simulink model "LoRaWAN_withoutGolay"  (R2021a)
settings: Solver=VariableStepAuto  StartTime=0.0  StopTime=1  RelTol=1e-3
libraries: commdigbbndcpm2 x2, commchan3 x1, commsink2 x1, commutil2 x1, commrflib2 x1, commrandsrc3 x1
settings Model: Creator=saivittalb  LastModifiedBy=saivittalb

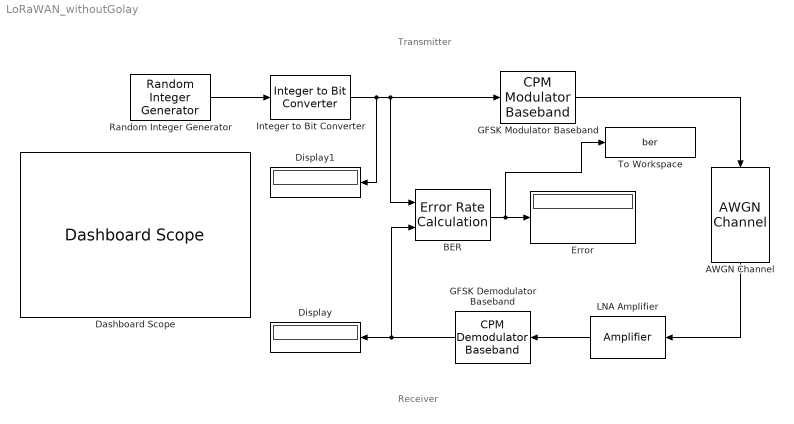
== system LoRaWAN_withoutGolay ==
  note: Transmitter
  note: Receiver
  AWGN Channel : commchan3/AWGN Channel  InputProcessing=Columns as channels (frame based)  seed=67  noiseMode="Signal to noise ratio  (Eb/No)"  EbNodB=10  EsNodB=10  SNRdB=1  bitsPerSym=2  Ps=1  Tsym=1e-6  variance=1
  BER : commsink2/Error Rate Calculation  N=72  st_delay=0  cp_mode=Entire frame  subframe=[]  PMode=Port  WsName=ErrorVec  RsMode2=off  stop=off  numErr=100  maxBits=1e6
  Dashboard Scope : DashboardScope
  Display : Display
  Display1 : Display
  Error : Display
  GFSK Demodulator Baseband : commdigbbndcpm2/CPM Demodulator Baseband  Mnum=2  outputType=Bit  mappingType=Binary  modIdx=0.5  pulseShape=Gaussian  BT=0.3  mainLobePulseLength=1  rollOff=0.2  pulseLength=1  preHistory=1  phaseOffset=1.5708  samplesPerSymbol=8  RateOptions=Enforce single-rate processing  traceBack=16  outDType=double
      settings: SourceProductBaseCode=CM
  GFSK Modulator Baseband : commdigbbndcpm2/CPM Modulator Baseband  Mnum=2  inputType=Bit  mappingType=Binary  modIdx=0.5  pulseShape=Gaussian  BT=0.3  mainLobePulseLength=1  rollOff=0.2  pulseLength=1  preHistory=1  phaseOffset=1.5708  samplesPerSymbol=8  RateOptions=Enforce single-rate processing  outDataType=double
      settings: SourceProductBaseCode=CM
  Integer to Bit Converter : commutil2/Integer to Bit Converter  nbits=2  signedInputValues=Unsigned  bitOrder=MSB first  outDtype=double
  LNA Amplifier : commrflib2/Amplifier  Model=Cubic polynomial  LinearGainDB=18  TOI_Type=IIP3  IIP3=Inf  OIP3=Inf  IP1dB=Inf  OP1dB=Inf  IPsat=Inf  OPsat=Inf  Table=[ -25, 5, -1; -10, 20, -2; 0, 27, 5; 5, 28, 12 ]  MagnitudeGainDB=0  Vsat=1  MagnitudeSmooth=2  PhaseGainRadian=-.45  PhaseSaturation=.88  PhaseSmooth=3.43  InputScaleDB=0  AmAmParameters=[ 2.1587, 1.1517 ]  AmPmParameters=[ 4.0033, 9.1040 ]  OutputScaleDB=0  SimulateUsing=Interpreted execution  IncludeNoise=on  NoiseType=Noise figure  NoiseTemperature=290  NoiseFigure=3  NoiseFactor=2  SeedSource=Auto  Seed=67987
      settings: SourceProductBaseCode=CM
  Random Integer Generator : commrandsrc3/Random Integer Generator  SetSize=2  SeedSource=Auto  Seed=0  SampleTime=1e-6  SamplesPerFrame=1024  OutputDataType=double  SimulateUsing=Interpreted execution
  To Workspace : ToWorkspace  VariableName=ber  SaveFormat=Timeseries  SampleTime=-1
  wires:
  GFSK Modulator Baseband/1 -> AWGN Channel/1
  AWGN Channel/1 -> LNA Amplifier/1
  LNA Amplifier/1 -> GFSK Demodulator Baseband/1
  GFSK Demodulator Baseband/1 -> BER/2, Display/1
  BER/1 -> To Workspace/1, Error/1
  Integer to Bit Converter/1 -> Display1/1, BER/1, GFSK Modulator Baseband/1
  Random Integer Generator/1 -> Integer to Bit Converter/1
